simulink library "fixpt_megmalib"  (Simulink 6.0)
settings: Solver=ode45  SolverMode=SingleTasking  StartTime=0.0  StopTime=10.0  RelTol=1e-3
undefined symbols (not defined in the file or in its folder): Bias1, Bias2, NumBits1, NumBits2, Slope1, Slope2
libraries: simulink x94, fixpt_megmaFuncBlkhidden1 x5, fixpt_megmalib x3
(part 1 of 3)
settings Model: Creator=krishnan  LastModifiedBy=andyb  ExtModeAutoUpdateStatusClock=off

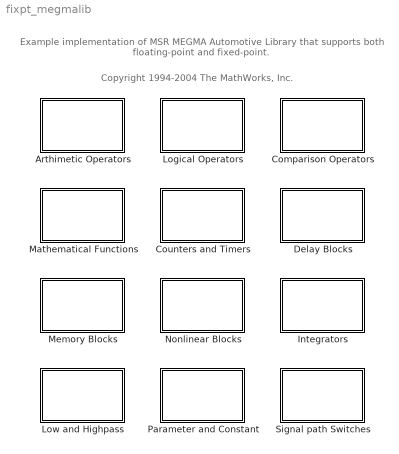
== system fixpt_megmalib ==
  note: Example implementation of MSR MEGMA Automotive Library
      | that supports both floating-point and fixed-point.
  note: Copyright 1994-2004 The MathWorks, Inc.
  Arthimetic Operators : Subsystem  PropExecContextAcrossSSBoundary=on
      mask Type: Arithmetic Blocks
      mask Display: disp('Arithmetic \n Operators')
  Comparison Operators : Subsystem  PropExecContextAcrossSSBoundary=on
      mask Type: Comparison
      mask Display: disp('Comparison \nOperators')
  Counters and Timers : Subsystem  PropExecContextAcrossSSBoundary=on
      mask Type: Count&Time
      mask Display: disp('Counters \n and Timers')
  Delay Blocks : Subsystem  PropExecContextAcrossSSBoundary=on
      mask Type: Count&Time
      mask Display: disp('Delay \n Blocks')
  Integrators : Subsystem  PropExecContextAcrossSSBoundary=on
      mask Type: Integrators
      mask Display: disp('Integrators')
  Logical Operators : Subsystem  PropExecContextAcrossSSBoundary=on
      mask Type: Logical
      mask Display: disp('Logical \n Operators')
  Low and Highpass : Subsystem  PropExecContextAcrossSSBoundary=on
      mask Type: LowAndHighPass
      mask Display: disp('Low and \n Highpass')
  Mathematical Functions : Subsystem  PropExecContextAcrossSSBoundary=on
      mask Type: Math
      mask Display: disp('Mathematical \n Functions')
  Memory Blocks : Subsystem  PropExecContextAcrossSSBoundary=on
      mask Type: Memory
      mask Display: disp('Memory \n Blocks')
  Nonlinear Blocks : Subsystem  PropExecContextAcrossSSBoundary=on
      mask Type: Nonlinear
      mask Display: disp('Nonlinear \n Blocks')
  Parameter and Constant : Subsystem  PropExecContextAcrossSSBoundary=on
      mask Type: ParameterAndConstant
      mask Display: disp('Parameter and \n Constant')
  Signal path Switches : Subsystem  PropExecContextAcrossSSBoundary=on
      mask Type: Switches
      mask Display: disp('Signal path \n Switches')

== system fixpt_megmalib/Arthimetic Operators ==
  note: Example implementation of MSR MEGMA Automotive Library
      | that supports both floating-point and fixed-point.
  note: Copyright 1994-2004 The MathWorks, Inc.
  Divide : Product  Inputs=*/  OutDataTypeMode=Specify via dialog  OutScaling=2^-10
  Gain : Gain  Gain=1.0  ParameterDataTypeMode=Specify via dialog  ParameterScaling=2^-15  OutDataTypeMode=Specify via dialog  OutScaling=2^-10
  Neg : simulink/Math Operations/Unary Minus  DoSatur=off
  Prod : Product  Inputs=***  OutDataTypeMode=Specify via dialog  OutScaling=2^-10
  Sum : Sum  Inputs=+++  OutDataTypeMode=Specify via dialog  OutScaling=2^-10

== system fixpt_megmalib/Comparison Operators ==
  note: Example implementation of MSR MEGMA Automotive Library
      | that supports both floating-point and fixed-point.
  note: Copyright 1994-2004 The MathWorks, Inc.
  Closed Interval : Subsystem  PropExecContextAcrossSSBoundary=on
      mask Type: MEGMA Interval Test Dynamic
      mask Description: Output is true, if the input value u is in the closed interval [MN,MX]
      mask Help: fpbhelp('closedinterval');
      mask Display: plot(0.25+0.75*[0 1],[0.2 0.2],0.25+0.75*[0.35 0.35],[0 1],0.25+0.75*[0 0.2 0.2 0.65 0.65 1],[0.25 0.25 0.75 0.75 0.25 0.25]);
  Equal : RelationalOperator  Operator===  LogicOutDataTypeMode=Specify via dialog  ZeroCross=off
  Greater Than : RelationalOperator  Operator=>  LogicOutDataTypeMode=Specify via dialog  ZeroCross=off
  Greater Than and Equal : RelationalOperator  LogicOutDataTypeMode=Specify via dialog  ZeroCross=off
  Left Open Interval : Subsystem  PropExecContextAcrossSSBoundary=on
      mask Type: MEGMA Interval Test Dynamic
      mask Description: Output is true, if the input value u is in the left open interval (MN,MX]
      mask Help: fpbhelp('leftopeninterval');
      mask Display:
      | plot(0.25+0.75*[0 1],[0.2 0.2],0.25+0.75*[0.35 0.35],[0 1],0.25+0.75*[0 0.2 0.2],...
      | [0.25 0.25 0.4],  0.25+0.75*[0.2 0.2 0.65 0.65 1],[0.6 0.75 0.75 0.25 0.25]);
  Less Than : RelationalOperator  Operator=<  LogicOutDataTypeMode=Specify via dialog  ZeroCross=off
  Less Than and Equal : RelationalOperator  Operator=<=  LogicOutDataTypeMode=Specify via dialog  ZeroCross=off
  Not equal : RelationalOperator  Operator=~=  LogicOutDataTypeMode=Specify via dialog  ZeroCross=off
  Open Interval : Subsystem  PropExecContextAcrossSSBoundary=on
      mask Type: MEGMA Interval Test Dynamic
      mask Description: Output is true, if the input value u is in the open interval (MN,MX)
      mask Help: fpbhelp('openinterval');
      mask Display:
      | plot(0.25+0.75*[0 1],[0.2 0.2],0.25+0.75*[0.35 0.35],[0 1],0.25+0.75*[0 0.2 0.2],...
      | [0.25 0.25 0.4],0.25+0.75*[0.2 0.2 0.65 0.65],[0.6 0.75 0.75 0.6],0.25+0.75*[0.65 0.65 1],[0.4 0.25 0.25])
  Right Open Interval : Subsystem  PropExecContextAcrossSSBoundary=on
      mask Type: MEGMA Interval Test Dynamic
      mask Description: Output is true, if the input value u is in the right open interval [MN,MX)
      mask Help: fpbhelp('rightopeninterval');
      mask Display:
      | plot(0.25+0.75*[0 1],[0.2 0.2],0.25+0.75*[0.35 0.35],[0 1],...
      | 0.25+0.75*[0 0.2 0.2 0.65 0.65],[0.25 0.25 0.75 0.75 0.6],   0.25+0.75*[0.65 0.65 1],[0.4 0.25 0.25]);

== system fixpt_megmalib/Counters and Timers ==
  note: Example implementation of MSR MEGMA Automotive Library
      | that supports both floating-point and fixed-point.
  note: Copyright 1994-2004 The MathWorks, Inc.
  CountDown ResetEnabled : Subsystem  PropExecContextAcrossSSBoundary=on
      mask Type: MEGMA CountDownResetEnabled
      mask Description: Outputs true, if the number of block evaluations sincethe last reset is less than the initial number of block evaluations IV
      mask Help: fpbhelp('countdownresetenabled');
      mask Display: plot(0.25+0.7/6*[0 1 1 2 2 3 3 4 4 6],0.15+0.7/3*[0 0 3 3 2 2 1 1 0 0])
  CountDown ResetTriggerEnabled : Subsystem  PropExecContextAcrossSSBoundary=on
      mask Type: MEGMA CountDownResetTriggerEnabled
      mask Description: Outputs true, if the number of block evaluations sincethe last reset is less than the initial number of block evaluations IV
      mask Help: fpbhelp('countdownresettriggerenabled');
      mask Display: plot(0.25+0.7/6*[0 1 1 2 2 3 3 4 4 6],0.15+0.7/3*[0 0 3 3 2 2 1 1 0 0])
  Counter ResetEnabled : Subsystem  PropExecContextAcrossSSBoundary=on  mask(MEGMA CounterResetEnabled){CounterBuiltInType=uint16}
      mask prompts: CounterBuiltInType "Output data type:"
      mask help: Counts up and outputs the number of block evaluations since the last reset
      mask init:
      | switch CounterBuiltInType
      | case 1
      | outDT = float('double');
      | case 2
      | outDT = float('single');
      | case 3
      | outDT = sint(8);
      | case 4
      | outDT = uint(8);
      | case 5
      | outDT = sint(16);
      | case 6
      | outDT = uint(16);
      | case 7
      | outDT = sint(32);
      | case 8
      | outDT = uint(32);
      | end
      mask Help: fpbhelp('counterresetenabled');
      mask StyleString: popup(double|single|int8|uint8|int16|uint16|int32|uint32)
      mask Display: plot(0.25+0.7/6*[0 1 1 2 2 3 3 4 4 5],0.15+0.7/4*[0 0 1 1 2 2 3 3 4 4])
  Counter ResetTriggerEnabled : Subsystem  PropExecContextAcrossSSBoundary=on  mask(MEGMA CounterResetEnabled){CounterBuiltInType=uint16}
      mask prompts: CounterBuiltInType "Output data type:"
      mask help: Counts up and outputs the number of block evaluations since the last reset
      mask init: same as fixpt_megmalib/Counters and Timers/Counter ResetEnabled
      mask Help: fpbhelp('counterresettriggerenabled');
      mask StyleString: popup(double|single|int8|uint8|int16|uint16|int32|uint32)
      mask Display: plot(0.25+0.7/6*[0 1 1 2 2 3 3 4 4 5],0.15+0.7/4*[0 0 1 1 2 2 3 3 4 4])
  StopWatch ResetEnabled : Subsystem  PropExecContextAcrossSSBoundary=on  mask(MEGMA StopWatchResetEnabled){StopWatchBuiltInType=uint16}
      mask prompts: StopWatchBuiltInType "Stop watch data type based on:"
      mask help: The block outputs the time since the system init or thelast reset
      mask init:
      | switch StopWatchBuiltInType
      | case 1
      | outDT = float('double');
      | case 2
      | outDT = float('single');
      | case 3
      | outDT = sint(8);
      | case 4
      | outDT = uint(8);
      | case 5
      | outDT = sint(16);
      | case 6
      | outDT = uint(16);
      | case 7
      | outDT = sint(32);
      | case 8
      | outDT = uint(32);
      | end
      | rad1 = 0.4;
      | rad2 = 0.3;
      | ntic = 12;
      | npts = ntic*2+1;
      | ang = linspace(0,2*pi,npts);
      | x = rad1*cos(ang);
      | y = rad1*sin(ang);
      | xx = zeros(2,ntic);
      | yy = xx;
      | for i = 1:ntic
      |  xx([1 2],i) = [rad1; rad2]*cos(2*pi/ntic*i);
      |  yy([1 2],i) = [rad1; rad2]*sin(2*pi/ntic*i);
      | end
      | dd = 0.1;
      | f45 = cos(pi/4);
      | d45 = dd  *f45;
      | r45 = rad2*f45;
      | xa = 0.6+[         d45 0 -d45 0    0   -r45+[0  0  0 dd]];
      | ya = 0.5+[(-rad2)+[d45 0  d45 0]   0    r45+[0 -dd 0 0 ]];
      mask Help: fpbhelp('stopwatchresetenabled');
      mask StyleString: popup(double|single|int8|uint8|int16|uint16|int32|uint32)
      mask Display: plot(x+0.6,y+0.5,xx+0.6,yy+0.5,xa,ya)
  StopWatch ResetTriggerEnabled : Subsystem  PropExecContextAcrossSSBoundary=on  mask(MEGMA StopWatchResetTriggerEnabled){StopWatchBuiltInType=uint16}
      mask prompts: StopWatchBuiltInType "Stop watch data type based on:"
      mask help: The block outputs the time since the system init or thelast reset
      mask init: same as fixpt_megmalib/Counters and Timers/StopWatch ResetEnabled
      mask Help: fpbhelp('stopwatchresettriggerenabled');
      mask StyleString: popup(double|single|int8|uint8|int16|uint16|int32|uint32)
      mask Display: plot(x+0.6,y+0.5,xx+0.6,yy+0.5,xa,ya)
  Timer ResetEnabled : Subsystem  PropExecContextAcrossSSBoundary=on
      mask Type: MEGMA TimerResetEnabled
      mask Description: The block indicates true, if the initial time IV has notpassed since the last reset of the block. Reset can onlybe performed, if the counter has run down to zero
      mask Help: fpbhelp('timerresetenabled');
      mask Display: plot(0.25+0.7/5*[0 1 1 4 5],0.15+0.7/1*[0 0 1 0 0])
  Timer ResetTriggerEnabled : Subsystem  PropExecContextAcrossSSBoundary=on
      mask Type: MEGMA TimerResetEnabled
      mask Description: The block indicates true, if the initial time IV has notpassed since the last reset of the block. Reset can onlybe performed, if the counter has run down to zero
      mask Help: fpbhelp('timerresettriggerenabled');
      mask Display: plot(0.25+0.7/5*[0 1 1 4 5],0.15+0.7/1*[0 0 1 0 0])
  Timer RetriggerReset TriggerEnabled : Subsystem  PropExecContextAcrossSSBoundary=on
      mask Type: MEGMA TimerRetriggerResetTriggerEnabled
      mask Description: The block indicates true, if the initial time IV has notpassed since the last reset of the block. Reset is alwayspossible and independent of the current timer value
      mask Help: fpbhelp('timerretriggerresettriggerenabled');
      mask Display: plot(0.25+0.7/8*[0 1 1 3 3 7 8],0.15+0.7/2*[0 0 2 1 2 0 0])
  Timer RetriggerResetEnabled : Subsystem  PropExecContextAcrossSSBoundary=on
      mask Type: MEGMA TimerRetriggerResetEnabled
      mask Description: The block indicates true, if the initial time IV has notpassed since the last reset of the block. Reset is alwayspossible and independent of the current timer value
      mask Help: fpbhelp('timerretriggerresetenabled');
      mask Display: plot(0.25+0.7/8*[0 1 1 3 3 7 8],0.15+0.7/2*[0 0 2 1 2 0 0])

== system fixpt_megmalib/Delay Blocks ==
  note: Example implementation of MSR MEGMA Automotive Library
      | that supports both floating-point and fixed-point.
  note: Copyright 1994-2004 The MathWorks, Inc.
  DelayResetEnabled : simulink/Additional Math & Discrete/Additional Discrete/Unit Delay Enabled Resettable External IC  tsamp=-1
  TurnOffDelaySample : Subsystem  PropExecContextAcrossSSBoundary=on  mask(MEGMA TurnOffDelaySample){CounterType=uint16}
      mask prompts: CounterType "State data type:"
      mask help: A falling edge of the input signal is delayed by n block evaluations
      mask init:
      | switch CounterType
      | case 1
      | outDT = uint(8);
      | case 2
      | outDT = uint(16);
      | case 3
      | outDT = uint(32);
      | end
      mask Help: fpbhelp('turnoffdelaysample');
      mask StyleString: popup(uint8|uint16|uint32)
      mask Display:
      | plot(0.25+0.7/6*[0 4 4 6],0.15+0.7/1*[1 1 0 0])
      | disp('n')
  TurnOffDelayTime : Subsystem  PropExecContextAcrossSSBoundary=on
      mask Type: MEGMA TurnOffDelayTime
      mask Description: A falling edge of the input signal u is delayed by the time T
      mask Help: fpbhelp('turnoffdelaytime');
      mask Display:
      | plot(0.25+0.7/6*[0 4 4 6],0.15+0.7/1*[1 1 0 0])
      | disp('T')
  TurnOnDelaySample : Subsystem  PropExecContextAcrossSSBoundary=on  mask(MEGMA TurnOffDelaySample){CounterType=uint16}
      mask prompts: CounterType "State data type:"
      mask help: A rising edge of the input signal is delayed by n block evaluations
      mask init:
      | switch CounterType
      | case 1
      | outDT = uint(8);
      | case 2
      | outDT = uint(16);
      | case 3
      | outDT = uint(32);
      | end
      mask Help: fpbhelp('turnondelaysample');
      mask StyleString: popup(uint8|uint16|uint32)
      mask Display:
      | plot(0.25+0.7/6*[0 4 4 6],0.15+0.7/1*[0 0 1 1])
      | disp('n')
  TurnOnDelayTime : Subsystem  PropExecContextAcrossSSBoundary=on
      mask Type: MEGMA TurnOnDelayTime
      mask Description: A rising edge of the input signal u is delayed by the time T
      mask Help: fpbhelp('turnondelaytime');
      mask Display:
      | plot(0.25+0.7/6*[0 4 4 6],0.15+0.7/1*[0 0 1 1])
      | disp('T')

== system fixpt_megmalib/Integrators ==
  note: Example implementation of MSR MEGMA Automotive Library
      | that supports both floating-point and fixed-point.
  note: Copyright 1994-2004 The MathWorks, Inc.
  Accumulator : Subsystem  PropExecContextAcrossSSBoundary=on
      mask Type: MEGMA Accumulator Reset Enabled Limited
      mask Description: Saves and outputs the limited sum of all input values u, starting with the reset value IV
      mask Help: fpbhelp('accumulator');
      mask Display: plot(0.3+0.65/6*[6 0 3 0 6],0.15+0.7/2*[0 0 1 2 2])
  IntegratorKReset EnabledLimited : Subsystem  PropExecContextAcrossSSBoundary=on
      mask Type: MEGMA Integrator K Reset Enabled Limited
      mask Description: A discrete time integrator with gain K and limitation of the integrator values to MN and MX.
      mask Help: fpbhelp('integratorkresetenabledlimited');
      mask Display:
      | plot(0.3+0.65/3*[0 0 3 0 2],0.05+0.9/1*[1 0 0 0 1])
      | text(0.6,0.4,'K')
  IntegratorTReset EnabledLimited : Subsystem  PropExecContextAcrossSSBoundary=on
      mask Type: MEGMA Integrator T Reset Enabled Limited
      mask Description: A discrete time integrator with gain 1/T and limitation of the integrator values to MN and MX.
      mask Help: fpbhelp('integratortresetenabledlimited');
      mask Display:
      | plot(0.3+0.65/3*[0 0 3 0 2],0.05+0.9/1*[1 0 0 0 1])
      | text(0.6,0.4,'T')

== system fixpt_megmalib/Logical Operators ==
  note: Example implementation of MSR MEGMA Automotive Library
      | that supports both floating-point and fixed-point.
  note: Copyright 1994-2004 The MathWorks, Inc.
  Logical AND : Logic  AllPortsSameDT=off  OutDataTypeMode=Specify via dialog
  Logical NOT : Logic  Operator=NOT  Inputs=1  AllPortsSameDT=off  OutDataTypeMode=Specify via dialog
  Logical OR : Logic  Operator=OR  AllPortsSameDT=off  OutDataTypeMode=Specify via dialog
  Logical XOR : Logic  Operator=XOR  Inputs=1  AllPortsSameDT=off  OutDataTypeMode=Specify via dialog

== system fixpt_megmalib/Low and Highpass ==
  note: Example implementation of MSR MEGMA Automotive Library
      | that supports both floating-point and fixed-point.
  note: Copyright 1994-2004 The MathWorks, Inc.
  DigitalLowPass ResetEnabled : Subsystem  PropExecContextAcrossSSBoundary=on
      mask Type: MEGMA DigitalLowPassResetEnabled
      mask Description:
      | A discrete time, fixed-point realization of a first order filter.
      | (1-p) z
      | ------
      | (z-p)
      | To manually adjust a setting such as scaling, look underthe mask to get at individual blocks. Scaling can alsobe set using the automatic scaling procedures
      mask Help: fpbhelp('digitallowpassresetenabled');
      mask Display:
      | plot([0.2,0.2],[0.2,0.8],[0.2 0.8],[0.2 0.2],...
      | [0.2 0.3 0.4 0.5 0.6 0.7 0.8 0.9],[0.2 0.3 0.4 0.45 0.5 0.52 0.52 0.52],...
      | [0.1,0.2],[0.54 0.54],[0.3 0.4],[0.54 0.54],[0.5 0.6],[0.54 0.54],...
      | [0.7 0.8],[0.54 0.54],[0.85 0.9],[0.54 0.54])
      | text(0.7,0.5,'m')
  HighPass TResetEnabled : Subsystem  PropExecContextAcrossSSBoundary=on
      mask Type: MEGMA HighPassTResetEnabled
      mask Description:
      | A discrete time, fixed-point realization of a first order filter.
      | TD s
      | ------
      | ( T s + 1 )
      | To manually adjust a setting such as scaling, look underthe mask to get at individual blocks. Scaling can alsobe set using the automatic scaling procedures
      mask Help: fpbhelp('highpasstresetenabled');
      mask Display:
      | plot([0.2,0.2],[0.2,0.8],[0.2 0.8],[0.2 0.2],...
      | [0.2 0.3 0.35 0.4 0.45 0.5 0.55 0.6 0.65],[0.6 0.45 0.4 0.35 0.32 0.3 0.26 0.25 0.22])
  LowPass KResetEnabled : Subsystem  PropExecContextAcrossSSBoundary=on
      mask Type: MEGMA LowPassKResetEnabled
      mask Description:
      | A discrete time, fixed-point realization of a first order filter.
      | K
      | ------
      | ( s + K )
      | To manually adjust a setting such as scaling, look underthe mask to get at individual blocks. Scaling can alsobe set using the automatic scaling procedures
      mask Help: fpbhelp('lowpasskresetenabled');
      mask Display:
      | plot([0.2,0.2],[0.2,0.8],[0.2 0.8],[0.2 0.2],...
      | [0.2 0.3 0.4 0.5 0.6 0.7 0.8 0.9],[0.2 0.3 0.4 0.45 0.5 0.52 0.52 0.52],...
      | [0.1,0.2],[0.54 0.54],[0.3 0.4],[0.54 0.54],[0.5 0.6],[0.54 0.54],...
      | [0.7 0.8],[0.54 0.54],[0.85 0.9],[0.54 0.54])
      | text(0.7,0.4,'K')
  LowPass TResetEnabled : Subsystem  PropExecContextAcrossSSBoundary=on
      mask Type: MEGMA LowPassTResetEnabled
      mask Description:
      | A discrete time, fixed-point realization of a first order filter.
      | 1
      | ------
      | ( Ts + 1 )
      | To manually adjust a setting such as scaling, look underthe mask to get at individual blocks. Scaling can alsobe set using the automatic scaling procedures
      mask Help: fpbhelp('lowpasstresetenabled');
      mask Display:
      | plot([0.2,0.2],[0.2,0.8],[0.2 0.8],[0.2 0.2],...
      | [0.2 0.3 0.4 0.5 0.6 0.7 0.8 0.9],[0.2 0.3 0.4 0.45 0.5 0.52 0.52 0.52],...
      | [0.1,0.2],[0.54 0.54],[0.3 0.4],[0.54 0.54],[0.5 0.6],[0.54 0.54],...
      | [0.7 0.8],[0.54 0.54],[0.85 0.9],[0.54 0.54])
      | text(0.7,0.4,'T')

== system fixpt_megmalib/Mathematical Functions ==
  note: Example implementation of MSR MEGMA Automotive Library
      | that supports both floating-point and fixed-point.
  note: Copyright 1994-2004 The MathWorks, Inc.
  Configurable Subsystem : Subsystem  BlockChoice=Sine  PropExecContextAcrossSSBoundary=on
      settings: AttributesFormatString=%<BlockChoice>  MemberBlocks=Floating point Sine,Sine
      settings: TemplateBlock=|
      | fixpt_megmaFuncBlkhidden1/Configurable
      | Subsystem
  Configurable Subsystem1 : Subsystem  BlockChoice=Cosine  PropExecContextAcrossSSBoundary=on
      settings: AttributesFormatString=%<BlockChoice>  MemberBlocks=Cosine,Floating point Cosine
      settings: TemplateBlock=|
      | fixpt_megmaFuncBlkhidden1/Configurable
      | Subsystem1
  Configurable Subsystem2 : Subsystem  BlockChoice=Tangent  PropExecContextAcrossSSBoundary=on
      settings: AttributesFormatString=%<BlockChoice>  MemberBlocks=Floating point tangent,Tangent
      settings: TemplateBlock=|
      | fixpt_megmaFuncBlkhidden1/Configurable
      | Subsystem2
  Configurable Subsystem3 : Subsystem  BlockChoice=Exponent  PropExecContextAcrossSSBoundary=on
      settings: AttributesFormatString=%<BlockChoice>  MemberBlocks=Exponent,Floating point Exponent
      settings: TemplateBlock=|
      | fixpt_megmaFuncBlkhidden1/Configurable
      | Subsystem3
  Configurable Subsystem4 : Subsystem  BlockChoice=Sqrt  PropExecContextAcrossSSBoundary=on
      settings: AttributesFormatString=%<BlockChoice>  MemberBlocks=Floating point sqrt,Sqrt
      settings: TemplateBlock=|
      | fixpt_megmaFuncBlkhidden1/Configurable
      | Subsystem4

== system fixpt_megmalib/Memory Blocks ==
  note: Example implementation of MSR MEGMA Automotive Library
      | that supports both floating-point and fixed-point.
  note: Copyright 1994-2004 The MathWorks, Inc.
  DeltaOneStep : Subsystem  PropExecContextAcrossSSBoundary=on
      mask Type: DeltaOneStep
      mask Description: A discrete time, fixed point realization of an input signal time difference
      mask Help: fpbhelp('deltaonestep');
      mask Display:
      | port_label('input',1,'u')
      | port_label('output',1,'y')
      | port_label('input',2,'R')
      | port_label('input',3,'IV')
      | plot([0.2 0.5],[0.3 0.7],[0.5 0.8],[0.7 0.3],[0.8 0.2],[0.3 0.3])
  DifferenceQuotient : Subsystem  PropExecContextAcrossSSBoundary=on
      mask Type: DifferenceQuotient
      mask Description: A discrete time, fixed point realization of the ratio of the input signal time difference by the sample time of the simulation
      mask Help: fpbhelp('differencequotient');
      mask Display:
      | port_label('input',1,'u')
      | port_label('input',2,'R')
      | port_label('input',3,'IV')
      | port_label('output',1,'y')
      | text(7,3,'T')
      | plot([0.2 0.3],[0.5 0.65],[0.3 0.4],[0.65 0.5],[0.2 0.4],[0.5 0.5],...
      | [0.25 0.55],[0.4 0.6],...
      | [0.3 0.4],[0.2 0.35],[0.4 0.5],[0.35 0.2],[0.3 0.5],[0.2 0.2],...
      | [0.6 0.6],[0.2 0.35],[0.55 0.65],[0.35 0.35])
  EdgeBi : Subsystem  PropExecContextAcrossSSBoundary=on
      mask Type: EdgeBi
      mask Description: Fixed point realization of the MEGMA EdgeBi block
      mask Help: fpbhelp('edgebi');
      mask Display:
      | port_label('input',1,'u')
      | port_label('input',2,'R')
      | port_label('input',3,'IV')
      | port_label('output',1,'y')
      | plot([0.3 0.5],[0.2 0.2],[0.5 0.5],[0.2 0.8],[0.5 0.7],[0.8 0.8],...
      | [0.4 0.5],[0.55 0.7],[0.5 0.6],[0.7 0.55],[0.4 0.6],[0.55 0.55],...
      | [0.4 0.5],[0.45 0.3],[0.5 0.6],[0.3 0.45],[0.4 0.6],[0.45 0.45])
  EdgeFalling : Subsystem  PropExecContextAcrossSSBoundary=on
      mask Type: MEGMA EdgeFalling
      mask Description: Fixed point realization of the MEGMA EdgeFalling block
      mask Help: fpbhelp('edgefalling');
      mask Display:
      | port_label('input',1,'u')
      | port_label('input',2,'R')
      | port_label('input',3,'IV')
      | port_label('output',1,'y')
      | plot([0.3 0.5],[0.8 0.8],[0.5 0.5],[0.8 0.2],[0.5 0.7],[0.2 0.2],...
      | [0.45 0.55],[0.6 0.6],[0.45 0.5],[0.6 0.4],[0.5 0.55],[0.4,0.6])
  EdgeRising : Subsystem  PropExecContextAcrossSSBoundary=on
      mask Type: MEGMA EdgeRising
      mask Description: Fixed point realization of the MEGMA EdgeRising block
      mask Help: fpbhelp('edgerising');
      mask Display:
      | port_label('input',1,'u')
      | port_label('input',2,'R')
      | port_label('input',3,'IV')
      | port_label('output',1,'y')
      | plot([0.3 0.5],[0.2 0.2],[0.5 0.5],[0.2 0.8],[0.5 0.7],[0.8 0.8],...
      | [0.4 0.6],[0.4 0.4],[0.4 0.5],[0.4 0.6],[0.5 0.6],[0.6 0.4])
  RSFlipFlop : Subsystem  PropExecContextAcrossSSBoundary=on
      mask Type: RSFlipFlop
      mask Description: RS Flip Flop block. Reset always dominates
      mask Help: fpbhelp('rsflipflop');
      mask Display:
      | port_label('input',2,'R')
      | port_label('input',1,'S')
      | port_label('output',1,'Q')
      | port_label('output',2,'!Q')
      | disp('FF')
  SampleAndHold ResetEnabled : Subsystem  PropExecContextAcrossSSBoundary=on
      mask Type: SampleAndHoldResetEnabled
      mask Description: Fixed point realization of the MEGMA sample and hold block
      mask Help: fpbhelp('sampleandholdresetenabled');
      mask Display:
      | disp('Sample\n and \nHold')
      | port_label('input',1,'u')
      | port_label('input',2,'R')
      | port_label('input',3,'IV')
      | port_label('input',4,'E')
  Unit Delay Enabled Resettable : simulink/Additional Math & Discrete/Additional Discrete/Unit Delay Enabled Resettable  vinit=0.0  tsamp=-1

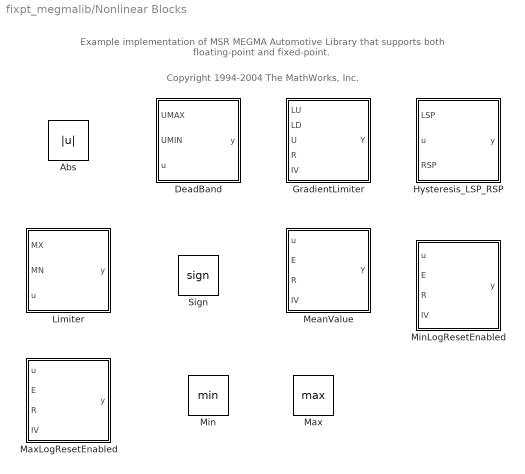
== system fixpt_megmalib/Nonlinear Blocks ==
  note: Example implementation of MSR MEGMA Automotive Library
      | that supports both floating-point and fixed-point.
  note: Copyright 1994-2004 The MathWorks, Inc.
  Abs : Abs  ZeroCross=off
  DeadBand : Subsystem  PropExecContextAcrossSSBoundary=on
      mask Type: MEGMA DeadBand
      mask Description: Dead Zone Dynamic
      mask Help: fpbhelp('deadband');
      mask Display: plot([0.2 0.8],[.5 .5],[.5 .5],[0.2 0.8],0.1+0.8*[0 .3 .7 1],0.1+0.8*[0.1 0.5 0.5 0.9])
  GradientLimiter : Subsystem  PropExecContextAcrossSSBoundary=on
      mask Type: MEGMA GradientLimiter
      mask Description: Limit rising and falling rates of signals. The output value is the input rate limited by LD or LU
      mask Help: fpbhelp('gradientlimiter');
      mask Display:
      | plot([0.2 0.8],[.5 .5],[.5 .5],[0.2 0.8],0.1+0.8*[0 .25 .75 1],0.1+0.8*[.25 .25 .75 .75]);
      | text(0.6,0.4,'GRD')
      | port_label('input',1,'LU')
      | port_label('input',2,'LD')
      | port_label('input',3,'u')
      | port_label('output',1,'y')
      | port_label('input',4,'R')
      | port_label('input',5,'IV')
  Hysteresis_LSP_RSP : Subsystem  PropExecContextAcrossSSBoundary=on
      mask Type: MEGMA Hysteresis_LSP_RSP
      mask Description: Falling edge and rising edge of the output value are atseparated switching points LSP and RSP
      mask Help: fpbhelp('hysteresis_lsp_rsp');
      mask Display: plot([0 .65 .65],[.3 .3 .8],[.35 .35 1],[.3 .8 .8]);
  Limiter : Subsystem  PropExecContextAcrossSSBoundary=on
      mask Type: MEGMA Limiter
      mask Description: Bound the range of the input. First evaluates the minimum of the input value and MX and then evaluates the maximum of this result and MN.
      mask Help: fpbhelp('limiter');
      mask Display: plot([0.2 0.8],[.5 .5],[.5 .5],[0.2 0.8],0.1+0.8*[0 .25 .75 1],0.1+0.8*[.25 .25 .75 .75]);
  Max : MinMax  Function=max  OutDataTypeMode=Specify via dialog  OutScaling=2^-10  ZeroCross=off
  MaxLogResetEnabled : Subsystem  PropExecContextAcrossSSBoundary=on
      mask Type: MEGMA MaxLogResetEnabled
      mask Description: The output value is the maxiimum value of all occurred input values u with respect to the initial value IV
      mask Help: fpbhelp('maxlogresetenabled');
      mask Display: disp('MaxLog')
  MeanValue : Subsystem  PropExecContextAcrossSSBoundary=on  mask(MEGMA Mean){nSample=4}
      mask prompts: nSample "Number of input sample to average"
      mask help: A discrete time, fixed point realization of an average
      mask Help: fpbhelp('meanvalue');
      mask Display:
      | plot([0.2 0.4],[0.8 0.8],[0.2 0.28],[0.8 0.7],[0.28 0.2],[0.7 0.6],[0.2 0.4], [0.6 0.6])
      | text(0.45,0.7,'Uk')
      | plot([0.15 0.5],[0.55 0.55])
      | text(0.3,0.45,'K')
  Min : MinMax  OutDataTypeMode=Specify via dialog  OutScaling=2^-10  ZeroCross=off
  MinLogResetEnabled : Subsystem  PropExecContextAcrossSSBoundary=on
      mask Type: MEGMA MinLogResetEnabled
      mask Description: The output value is the minimum value of all occurred input values u with respect to the initial value IV
      mask Help: fpbhelp('minlogresetenabled');
      mask Display: disp('MinLog')
  Sign : Signum  ZeroCross=off

== system fixpt_megmalib/Parameter and Constant ==
  note: Example implementation of MSR MEGMA Automotive Library
      | that supports both floating-point and fixed-point.
  note: Copyright 1994-2004 The MathWorks, Inc.
  ConstReal : Constant  Value=0.0  OutDataTypeMode=Specify via dialog  ConRadixGroup=Best Precision: Vector-wise  OutScaling=2^-10
  Parameter1D Index : Lookup  DialogController=Simulink.DDGSource  InputValues=-5:5  OutputValues=tanh([-5:5])  LookUpMeth=Use Input Below  OutDataTypeMode=Specify via dialog  OutScaling=2^-10
  Parameter1D Interpolation : Lookup  DialogController=Simulink.DDGSource  InputValues=-5:5  OutputValues=tanh([-5:5])  LookUpMeth=Interpolation-Use End Values  OutDataTypeMode=Specify via dialog  OutScaling=2^-10
  Parameter2D Index : Lookup2D  DialogController=Simulink.DDGSource  RowIndex=[1:3]  ColumnIndex=[1:3]  OutputValues=[4 5 6;16 19 20;10 18 23]  LookUpMeth=Use Input Below  OutDataTypeMode=Specify via dialog  OutScaling=2^-10
  Parameter2D Interpolation : Lookup2D  DialogController=Simulink.DDGSource  RowIndex=[1:3]  ColumnIndex=[1:3]  OutputValues=[4 5 6;16 19 20;10 18 23]  LookUpMeth=Interpolation-Use End Values  OutDataTypeMode=Specify via dialog  OutScaling=2^-10

== system fixpt_megmalib/Signal path Switches ==
  note: Example implementation of MSR MEGMA Automotive Library
      | that supports both floating-point and fixed-point.
  note: Copyright 1994-2004 The MathWorks, Inc.
  MultiPort Switch : MultiPortSwitch  Inputs=3
  Switch : Switch  Threshold=1  ZeroCross=off

== system fixpt_megmalib/Comparison Operators/Closed Interval ==
  MX : Inport  LatchInput=off
  MN : Inport  Port=2  LatchInput=off
  u : Inport  Port=3  LatchInput=off
  Interval Test Dynamic : simulink/Logic and Bit Operations/Interval Test Dynamic  IntervalClosedRight=on  IntervalClosedLeft=on  LogicOutDataTypeMode=boolean
  y : Outport
  wires:
  Interval Test Dynamic/1 -> y/1
  u/1 -> Interval Test Dynamic/2
  MX/1 -> Interval Test Dynamic/1
  MN/1 -> Interval Test Dynamic/3

== system fixpt_megmalib/Comparison Operators/Left Open Interval ==
  MX : Inport  LatchInput=off
  MN : Inport  Port=2  LatchInput=off
  u : Inport  Port=3  LatchInput=off
  Interval Test Dynamic : simulink/Logic and Bit Operations/Interval Test Dynamic  IntervalClosedRight=on  IntervalClosedLeft=off  LogicOutDataTypeMode=boolean
  y : Outport
  wires:
  Interval Test Dynamic/1 -> y/1
  u/1 -> Interval Test Dynamic/2
  MN/1 -> Interval Test Dynamic/3
  MX/1 -> Interval Test Dynamic/1

== system fixpt_megmalib/Comparison Operators/Open Interval ==
  MX : Inport  LatchInput=off
  MN : Inport  Port=2  LatchInput=off
  u : Inport  Port=3  LatchInput=off
  Interval Test Dynamic : simulink/Logic and Bit Operations/Interval Test Dynamic  IntervalClosedRight=off  IntervalClosedLeft=off  LogicOutDataTypeMode=boolean
  y : Outport
  wires:
  Interval Test Dynamic/1 -> y/1
  u/1 -> Interval Test Dynamic/2
  MN/1 -> Interval Test Dynamic/3
  MX/1 -> Interval Test Dynamic/1

== system fixpt_megmalib/Comparison Operators/Right Open Interval ==
  MX : Inport  LatchInput=off
  MN : Inport  Port=2  LatchInput=off
  u : Inport  Port=3  LatchInput=off
  Interval Test Dynamic : simulink/Logic and Bit Operations/Interval Test Dynamic  IntervalClosedRight=off  IntervalClosedLeft=on  LogicOutDataTypeMode=boolean
  y : Outport
  wires:
  Interval Test Dynamic/1 -> y/1
  u/1 -> Interval Test Dynamic/2
  MN/1 -> Interval Test Dynamic/3
  MX/1 -> Interval Test Dynamic/1

== system fixpt_megmalib/Counters and Timers/CountDown ResetEnabled ==
  E : Inport  LatchInput=off
  R : Inport  Port=2  LatchInput=off
  IV : Inport  Port=3  LatchInput=off
  Decrement To Zero : simulink/Additional Math & Discrete/Additional Math: Increment - Decrement/Decrement To Zero
  Positive : simulink/Logic and Bit Operations/Compare To Zero  relop=>  LogicOutDataTypeMode=uint8
  ResetEnabledState : Subsystem  PropExecContextAcrossSSBoundary=on
  y : Outport
  wires:
  E/1 -> ResetEnabledState/1(E)  "Enable"
  Positive/1 -> y/1
  IV/1 -> ResetEnabledState/3(IV)  "Initial Value"
  Decrement To Zero/1 -> ResetEnabledState/4(Xcalc)
  ResetEnabledState/2(Xold) -> Decrement To Zero/1  "Xold"
  ResetEnabledState/1(Xnew) -> Positive/1  "Xnew"
  R/1 -> ResetEnabledState/2(R)  "Reset"

== system fixpt_megmalib/Counters and Timers/CountDown ResetTriggerEnabled ==
  E : Inport  LatchInput=off
  RT : Inport  Port=2  LatchInput=off
  IV : Inport  Port=3  LatchInput=off
  Decrement To Zero : simulink/Additional Math & Discrete/Additional Math: Increment - Decrement/Decrement To Zero
  Detect Increase : simulink/Logic and Bit Operations/Detect Increase  vinit=0.0
  Positive : simulink/Logic and Bit Operations/Compare To Zero  relop=>  LogicOutDataTypeMode=uint8
  ResetEnabledState : Subsystem  PropExecContextAcrossSSBoundary=on
  y : Outport
  wires:
  Detect Increase/1 -> ResetEnabledState/2(R)  "Reset"
  RT/1 -> Detect Increase/1  "ResetTrigger"
  ResetEnabledState/1(Xnew) -> Positive/1  "Xnew"
  ResetEnabledState/2(Xold) -> Decrement To Zero/1  "Xold"
  Decrement To Zero/1 -> ResetEnabledState/4(Xcalc)
  IV/1 -> ResetEnabledState/3(IV)  "Initial Value"
  Positive/1 -> y/1
  E/1 -> ResetEnabledState/1(E)  "Enable"

== system fixpt_megmalib/Counters and Timers/Counter ResetEnabled ==
  E : Inport  LatchInput=off
  R : Inport  Port=2  LatchInput=off
  Ground3 : Ground  Orientation=left
  Ground4 : Ground  Orientation=left
  Increment Real World : simulink/Additional Math & Discrete/Additional Math: Increment - Decrement/Increment Real World
  ResetEnabledState : Subsystem  PropExecContextAcrossSSBoundary=on
  Set Ground Data Type : simulink/Signal Attributes/Data Type Propagation  Orientation=left  PropDataTypeMode=Specify via dialog  PropDataType=outDT  IfRefDouble=double  IfRefSingle=single  IsSigned=IsSigned1 or IsSigned2  NumBitsBase=max([NumBits1 NumBits2])  NumBitsMult=1  NumBitsAdd=0  NumBitsAllowFinal=1:128  PropScalingMode=Specify via dialog  PropScaling=1  ValuesUsedBestPrec=[5 -7]  SlopeBase=min([Slope1 Slope2])  SlopeMult=1  SlopeAdd=0  BiasBase=Bias1  BiasMult=1  BiasAdd=0
  y : Outport
  wires:
  Ground3/1 -> Set Ground Data Type/3, ResetEnabledState/3(IV)  "Initial Value"
  Ground4/1 -> Set Ground Data Type/1, Set Ground Data Type/2
  E/1 -> ResetEnabledState/1(E)  "Enable"
  Increment Real World/1 -> ResetEnabledState/4(Xcalc)
  ResetEnabledState/2(Xold) -> Increment Real World/1  "Xold"
  ResetEnabledState/1(Xnew) -> y/1  "Xnew"
  R/1 -> ResetEnabledState/2(R)  "Reset"

== system fixpt_megmalib/Counters and Timers/Counter ResetTriggerEnabled ==
  E : Inport  LatchInput=off
  RT : Inport  Port=2  LatchInput=off
  Detect Increase : simulink/Logic and Bit Operations/Detect Increase  vinit=0.0
  Ground1 : Ground  Orientation=left
  Ground2 : Ground  Orientation=left
  Increment Real World : simulink/Additional Math & Discrete/Additional Math: Increment - Decrement/Increment Real World
  ResetEnabledState : Subsystem  PropExecContextAcrossSSBoundary=on
  Set Ground Data Type : simulink/Signal Attributes/Data Type Propagation  Orientation=left  PropDataTypeMode=Specify via dialog  PropDataType=outDT  IfRefDouble=double  IfRefSingle=single  IsSigned=IsSigned1 or IsSigned2  NumBitsBase=max([NumBits1 NumBits2])  NumBitsMult=1  NumBitsAdd=0  NumBitsAllowFinal=1:128  PropScalingMode=Specify via dialog  PropScaling=1  ValuesUsedBestPrec=[5 -7]  SlopeBase=min([Slope1 Slope2])  SlopeMult=1  SlopeAdd=0  BiasBase=Bias1  BiasMult=1  BiasAdd=0
  y : Outport
  wires:
  RT/1 -> Detect Increase/1  "ResetTrigger"
  Detect Increase/1 -> ResetEnabledState/2(R)  "Reset"
  ResetEnabledState/1(Xnew) -> y/1  "Xnew"
  ResetEnabledState/2(Xold) -> Increment Real World/1  "Xold"
  Increment Real World/1 -> ResetEnabledState/4(Xcalc)
  Ground1/1 -> Set Ground Data Type/3, ResetEnabledState/3(IV)  "Initial Value"
  E/1 -> ResetEnabledState/1(E)  "Enable"
  Ground2/1 -> Set Ground Data Type/1, Set Ground Data Type/2

== system fixpt_megmalib/Counters and Timers/StopWatch ResetEnabled ==
  E : Inport  LatchInput=off
  R : Inport  Port=2  LatchInput=off
  FixPt Sample Time Math : simulink/Math Operations/Weighted Sample Time Math  TsampMathOp=*  weightValue=1.0  TsampMathImp=Online Calculations  DoSatur=off
  Ground3 : Ground  Orientation=left
  Ground4 : Ground  Orientation=left
  Increment Real World : simulink/Additional Math & Discrete/Additional Math: Increment - Decrement/Increment Real World
  ResetEnabledState : Subsystem  PropExecContextAcrossSSBoundary=on
  Set Ground Data Type : simulink/Signal Attributes/Data Type Propagation  Orientation=left  PropDataTypeMode=Specify via dialog  PropDataType=outDT  IfRefDouble=double  IfRefSingle=single  IsSigned=IsSigned1 or IsSigned2  NumBitsBase=max([NumBits1 NumBits2])  NumBitsMult=1  NumBitsAdd=0  NumBitsAllowFinal=1:128  PropScalingMode=Specify via dialog  PropScaling=1  ValuesUsedBestPrec=[5 -7]  SlopeBase=min([Slope1 Slope2])  SlopeMult=1  SlopeAdd=0  BiasBase=Bias1  BiasMult=1  BiasAdd=0
  y : Outport
  wires:
  Increment Real World/1 -> ResetEnabledState/4(Xcalc)
  ResetEnabledState/2(Xold) -> Increment Real World/1  "Xold"
  Ground4/1 -> Set Ground Data Type/2, Set Ground Data Type/1
  FixPt Sample Time Math/1 -> y/1
  ResetEnabledState/1(Xnew) -> FixPt Sample Time Math/1  "Xnew"
  R/1 -> ResetEnabledState/2(R)  "Reset"
  E/1 -> ResetEnabledState/1(E)  "Enable"
  Ground3/1 -> Set Ground Data Type/3, ResetEnabledState/3(IV)  "Initial Value"

== system fixpt_megmalib/Counters and Timers/StopWatch ResetTriggerEnabled ==
  E : Inport  LatchInput=off
  RT : Inport  Port=2  LatchInput=off
  Detect Increase : simulink/Logic and Bit Operations/Detect Increase  vinit=0.0
  FixPt Sample Time Math : simulink/Math Operations/Weighted Sample Time Math  TsampMathOp=*  weightValue=1.0  TsampMathImp=Online Calculations  DoSatur=off
  Ground3 : Ground  Orientation=left
  Ground4 : Ground  Orientation=left
  Increment Real World : simulink/Additional Math & Discrete/Additional Math: Increment - Decrement/Increment Real World
  ResetEnabledState : Subsystem  PropExecContextAcrossSSBoundary=on
  Set Ground Data Type : simulink/Signal Attributes/Data Type Propagation  Orientation=left  PropDataTypeMode=Specify via dialog  PropDataType=outDT  IfRefDouble=double  IfRefSingle=single  IsSigned=IsSigned1 or IsSigned2  NumBitsBase=max([NumBits1 NumBits2])  NumBitsMult=1  NumBitsAdd=0  NumBitsAllowFinal=1:128  PropScalingMode=Specify via dialog  PropScaling=1  ValuesUsedBestPrec=[5 -7]  SlopeBase=min([Slope1 Slope2])  SlopeMult=1  SlopeAdd=0  BiasBase=Bias1  BiasMult=1  BiasAdd=0
  y : Outport
  wires:
  RT/1 -> Detect Increase/1  "ResetTrigger"
  Ground3/1 -> Set Ground Data Type/3, ResetEnabledState/3(IV)  "Initial Value"
  E/1 -> ResetEnabledState/1(E)  "Enable"
  Detect Increase/1 -> ResetEnabledState/2(R)  "Reset"
  ResetEnabledState/1(Xnew) -> FixPt Sample Time Math/1  "Xnew"
  FixPt Sample Time Math/1 -> y/1
  Ground4/1 -> Set Ground Data Type/1, Set Ground Data Type/2
  ResetEnabledState/2(Xold) -> Increment Real World/1  "Xold"
  Increment Real World/1 -> ResetEnabledState/4(Xcalc)

== system fixpt_megmalib/Counters and Timers/Timer ResetEnabled ==
  E : Inport  LatchInput=off
  R : Inport  Port=2  LatchInput=off
  IV : Inport  Port=3  LatchInput=off
  Decrement Time To Zero : simulink/Additional Math & Discrete/Additional Math: Increment - Decrement/Decrement Time To Zero
  FixPt Logical Operator : Logic  AllPortsSameDT=off  OutDataTypeMode=Specify via dialog
  Nonpositive : simulink/Logic and Bit Operations/Compare To Zero  relop=<=  LogicOutDataTypeMode=uint8
  Positive : simulink/Logic and Bit Operations/Compare To Zero  relop=>  LogicOutDataTypeMode=uint8
  ResetEnabledState : Subsystem  PropExecContextAcrossSSBoundary=on
  y : Outport
  wires:
  Nonpositive/1 -> FixPt Logical Operator/2
  FixPt Logical Operator/1 -> ResetEnabledState/2(R)
  R/1 -> FixPt Logical Operator/1  "Reset"
  ResetEnabledState/1(Xnew) -> Positive/1  "Xnew"
  ResetEnabledState/2(Xold) -> Decrement Time To Zero/1, Nonpositive/1  "Xold"
  Decrement Time To Zero/1 -> ResetEnabledState/4(Xcalc)
  IV/1 -> ResetEnabledState/3(IV)  "Initial Value"
  Positive/1 -> y/1
  E/1 -> ResetEnabledState/1(E)  "Enable"

== system fixpt_megmalib/Counters and Timers/Timer ResetTriggerEnabled ==
  E : Inport  LatchInput=off
  RT : Inport  Port=2  LatchInput=off
  IV : Inport  Port=3  LatchInput=off
  Decrement Time To Zero : simulink/Additional Math & Discrete/Additional Math: Increment - Decrement/Decrement Time To Zero
  Detect Increase : simulink/Logic and Bit Operations/Detect Increase  vinit=0.0
  FixPt Logical Operator : Logic  AllPortsSameDT=off  OutDataTypeMode=Specify via dialog
  Nonpositive : simulink/Logic and Bit Operations/Compare To Zero  relop=<=  LogicOutDataTypeMode=uint8
  Positive : simulink/Logic and Bit Operations/Compare To Zero  relop=>  LogicOutDataTypeMode=uint8
  ResetEnabledState : Subsystem  PropExecContextAcrossSSBoundary=on
  y : Outport
  wires:
  RT/1 -> Detect Increase/1  "ResetTrigger"
  E/1 -> ResetEnabledState/1(E)  "Enable"
  Positive/1 -> y/1
  IV/1 -> ResetEnabledState/3(IV)  "Initial Value"
  Decrement Time To Zero/1 -> ResetEnabledState/4(Xcalc)
  ResetEnabledState/2(Xold) -> Decrement Time To Zero/1, Nonpositive/1  "Xold"
  ResetEnabledState/1(Xnew) -> Positive/1  "Xnew"
  Detect Increase/1 -> FixPt Logical Operator/1  "Reset"
  FixPt Logical Operator/1 -> ResetEnabledState/2(R)
  Nonpositive/1 -> FixPt Logical Operator/2

== system fixpt_megmalib/Counters and Timers/Timer RetriggerReset TriggerEnabled ==
  E : Inport  LatchInput=off
  RT : Inport  Port=2  LatchInput=off
  IV : Inport  Port=3  LatchInput=off
  Decrement Time To Zero : simulink/Additional Math & Discrete/Additional Math: Increment - Decrement/Decrement Time To Zero
  Detect Increase : simulink/Logic and Bit Operations/Detect Increase  vinit=0.0
  Positive : simulink/Logic and Bit Operations/Compare To Zero  relop=>  LogicOutDataTypeMode=uint8
  ResetEnabledState : Subsystem  PropExecContextAcrossSSBoundary=on
  y : Outport
  wires:
  RT/1 -> Detect Increase/1  "ResetTrigger"
  Detect Increase/1 -> ResetEnabledState/2(R)  "Reset"
  ResetEnabledState/1(Xnew) -> Positive/1  "Xnew"
  ResetEnabledState/2(Xold) -> Decrement Time To Zero/1  "Xold"
  Decrement Time To Zero/1 -> ResetEnabledState/4(Xcalc)
  IV/1 -> ResetEnabledState/3(IV)  "Initial Value"
  Positive/1 -> y/1
  E/1 -> ResetEnabledState/1(E)  "Enable"

== system fixpt_megmalib/Counters and Timers/Timer RetriggerResetEnabled ==
  E : Inport  LatchInput=off
  R : Inport  Port=2  LatchInput=off
  IV : Inport  Port=3  LatchInput=off
  Decrement Time To Zero : simulink/Additional Math & Discrete/Additional Math: Increment - Decrement/Decrement Time To Zero
  Positive : simulink/Logic and Bit Operations/Compare To Zero  relop=>  LogicOutDataTypeMode=uint8
  ResetEnabledState : Subsystem  PropExecContextAcrossSSBoundary=on
  y : Outport
  wires:
  E/1 -> ResetEnabledState/1(E)  "Enable"
  Positive/1 -> y/1
  IV/1 -> ResetEnabledState/3(IV)  "Initial Value"
  Decrement Time To Zero/1 -> ResetEnabledState/4(Xcalc)
  ResetEnabledState/2(Xold) -> Decrement Time To Zero/1  "Xold"
  ResetEnabledState/1(Xnew) -> Positive/1  "Xnew"
  R/1 -> ResetEnabledState/2(R)  "Reset"

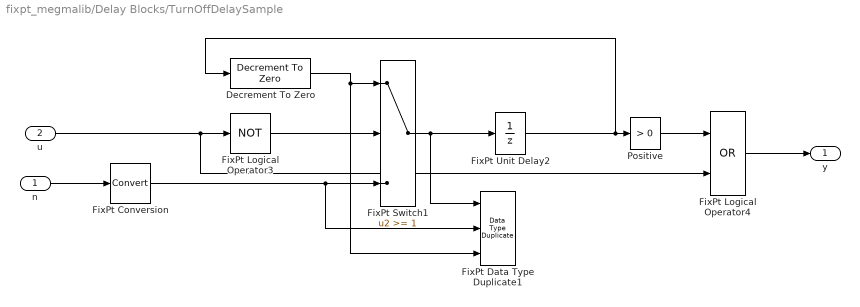
== system fixpt_megmalib/Delay Blocks/TurnOffDelaySample ==
  n : Inport  LatchInput=off
  u : Inport  Port=2  LatchInput=off
  Decrement To Zero : simulink/Additional Math & Discrete/Additional Math: Increment - Decrement/Decrement To Zero
  FixPt Conversion : DataTypeConversion  OutDataTypeMode=Specify via dialog  OutDataType=outDT  OutScaling=1  RndMeth=Nearest  SaturateOnIntegerOverflow=on
  FixPt Data Type Duplicate1 : simulink/Signal Attributes/Data Type Duplicate  NumInputPorts=3
  FixPt Logical Operator3 : Logic  Operator=NOT  Inputs=1  AllPortsSameDT=off  OutDataTypeMode=Specify via dialog
  FixPt Logical Operator4 : Logic  Operator=OR  AllPortsSameDT=off  OutDataTypeMode=Specify via dialog
  FixPt Switch1 : Switch  Threshold=1  ZeroCross=off
  FixPt Unit Delay2 : UnitDelay  X0=0.0  SampleTime=-1
  Positive : simulink/Logic and Bit Operations/Compare To Zero  relop=>  LogicOutDataTypeMode=uint8
  y : Outport
  wires:
  FixPt Logical Operator4/1 -> y/1
  Positive/1 -> FixPt Logical Operator4/1
  FixPt Conversion/1 -> FixPt Data Type Duplicate1/2, FixPt Switch1/3
  FixPt Unit Delay2/1 -> Decrement To Zero/1, Positive/1
  Decrement To Zero/1 -> FixPt Data Type Duplicate1/3, FixPt Switch1/1
  FixPt Switch1/1 -> FixPt Data Type Duplicate1/1, FixPt Unit Delay2/1
  FixPt Logical Operator3/1 -> FixPt Switch1/2
  u/1 -> FixPt Logical Operator4/2, FixPt Logical Operator3/1
  n/1 -> FixPt Conversion/1

== system fixpt_megmalib/Delay Blocks/TurnOffDelayTime ==
  T : Inport  LatchInput=off
  u : Inport  Port=2  LatchInput=off
  Decrement Time To Zero : simulink/Additional Math & Discrete/Additional Math: Increment - Decrement/Decrement Time To Zero
  FixPt Data Type Duplicate : simulink/Signal Attributes/Data Type Duplicate  NumInputPorts=3
  FixPt Logical Operator1 : Logic  Operator=NOT  Inputs=1  AllPortsSameDT=off  OutDataTypeMode=Specify via dialog
  FixPt Logical Operator2 : Logic  Operator=OR  AllPortsSameDT=off  OutDataTypeMode=Specify via dialog
  FixPt Switch3 : Switch  Threshold=1  ZeroCross=off
  FixPt Unit Delay1 : UnitDelay  X0=0.0  SampleTime=-1
  Positive : simulink/Logic and Bit Operations/Compare To Zero  relop=>  LogicOutDataTypeMode=uint8
  y : Outport
  wires:
  FixPt Logical Operator2/1 -> y/1
  Positive/1 -> FixPt Logical Operator2/1
  T/1 -> FixPt Data Type Duplicate/2, FixPt Switch3/3
  FixPt Unit Delay1/1 -> Decrement Time To Zero/1, Positive/1
  Decrement Time To Zero/1 -> FixPt Data Type Duplicate/3, FixPt Switch3/1
  FixPt Switch3/1 -> FixPt Data Type Duplicate/1, FixPt Unit Delay1/1
  FixPt Logical Operator1/1 -> FixPt Switch3/2
  u/1 -> FixPt Logical Operator2/2, FixPt Logical Operator1/1

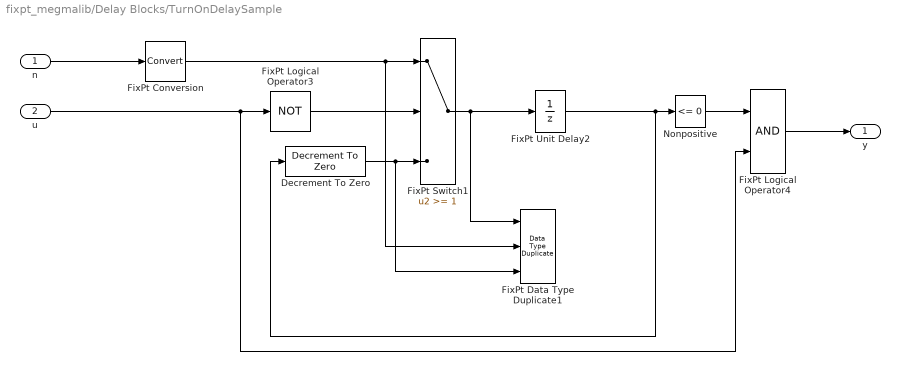
== system fixpt_megmalib/Delay Blocks/TurnOnDelaySample ==
  n : Inport  LatchInput=off
  u : Inport  Port=2  LatchInput=off
  Decrement To Zero : simulink/Additional Math & Discrete/Additional Math: Increment - Decrement/Decrement To Zero
  FixPt Conversion : DataTypeConversion  OutDataTypeMode=Specify via dialog  OutDataType=outDT  OutScaling=1  RndMeth=Nearest  SaturateOnIntegerOverflow=on
  FixPt Data Type Duplicate1 : simulink/Signal Attributes/Data Type Duplicate  NumInputPorts=3
  FixPt Logical Operator3 : Logic  Operator=NOT  Inputs=1  AllPortsSameDT=off  OutDataTypeMode=Specify via dialog
  FixPt Logical Operator4 : Logic  AllPortsSameDT=off  OutDataTypeMode=Specify via dialog
  FixPt Switch1 : Switch  Threshold=1  ZeroCross=off
  FixPt Unit Delay2 : UnitDelay  X0=0.0  SampleTime=-1
  Nonpositive : simulink/Logic and Bit Operations/Compare To Zero  relop=<=  LogicOutDataTypeMode=uint8
  y : Outport
  wires:
  n/1 -> FixPt Conversion/1
  FixPt Logical Operator4/1 -> y/1
  Nonpositive/1 -> FixPt Logical Operator4/1
  FixPt Conversion/1 -> FixPt Switch1/1, FixPt Data Type Duplicate1/2
  FixPt Unit Delay2/1 -> Decrement To Zero/1, Nonpositive/1
  Decrement To Zero/1 -> FixPt Switch1/3, FixPt Data Type Duplicate1/3
  FixPt Switch1/1 -> FixPt Data Type Duplicate1/1, FixPt Unit Delay2/1
  FixPt Logical Operator3/1 -> FixPt Switch1/2
  u/1 -> FixPt Logical Operator4/2, FixPt Logical Operator3/1

== system fixpt_megmalib/Delay Blocks/TurnOnDelayTime ==
  T : Inport  LatchInput=off
  u : Inport  Port=2  LatchInput=off
  Decrement Time To Zero : simulink/Additional Math & Discrete/Additional Math: Increment - Decrement/Decrement Time To Zero
  FixPt Data Type Duplicate1 : simulink/Signal Attributes/Data Type Duplicate  NumInputPorts=3
  FixPt Logical Operator3 : Logic  Operator=NOT  Inputs=1  AllPortsSameDT=off  OutDataTypeMode=Specify via dialog
  FixPt Logical Operator4 : Logic  AllPortsSameDT=off  OutDataTypeMode=Specify via dialog
  FixPt Switch1 : Switch  Threshold=1  ZeroCross=off
  FixPt Unit Delay2 : UnitDelay  X0=0.0  SampleTime=-1
  Nonpositive : simulink/Logic and Bit Operations/Compare To Zero  relop=<=  LogicOutDataTypeMode=uint8
  y : Outport
  wires:
  FixPt Logical Operator4/1 -> y/1
  Nonpositive/1 -> FixPt Logical Operator4/1
  T/1 -> FixPt Switch1/1, FixPt Data Type Duplicate1/2
  FixPt Unit Delay2/1 -> Decrement Time To Zero/1, Nonpositive/1
  Decrement Time To Zero/1 -> FixPt Switch1/3, FixPt Data Type Duplicate1/3
  FixPt Switch1/1 -> FixPt Data Type Duplicate1/1, FixPt Unit Delay2/1
  FixPt Logical Operator3/1 -> FixPt Switch1/2
  u/1 -> FixPt Logical Operator4/2, FixPt Logical Operator3/1
